simulink model "SingleTankOnOffControl_sim"  (R2021a)
settings: Solver=FixedStepAuto  StartTime=0.0  StopTime=40  FixedStep=0.1  RelTol=1e-3
InitFcn:
  | clearvars;
  | load('singletank_parameters.mat')
StopFcn:
  | plot_results
values from neighbouring files (symbols this model uses):
  params_single =     [singletank_parameters.mat]
libraries: simulink x1
settings Model: Creator=ksto036  LastModifiedBy=bl4ck
settings SolverCC: AlgebraicLoopSolver=TrustRegion
settings DataIOCC: SaveOutput=off  SignalLogging=off  DSMLogging=off  SaveTime=off  ReturnWorkspaceOutputs=off
settings DebuggingCC: SFMachineParentedDataDiag=warning

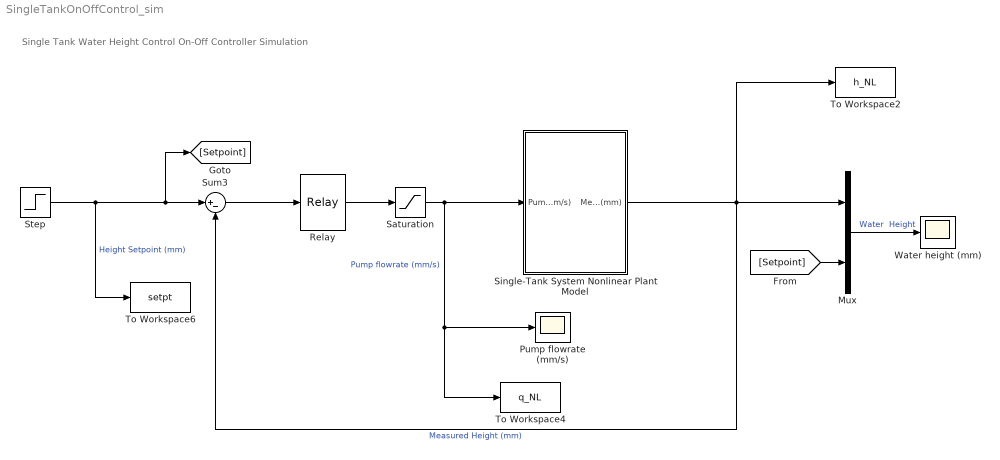
== system SingleTankOnOffControl_sim ==
  note: Single Tank Water Height Control
      | On-Off Controller
      | Simulation
  " Single-Tank System Nonlinear Plant Model" : Subsystem
      mask Display: image('$imagefile'); % Use "Edit Image" on toolstrip to change.
  Mux : Mux  Inputs=2
  Pump flowrate (mm/s) : Scope
  Relay : Relay  OnSwitchValue=3  OffSwitchValue=-3  OnOutputValue=params_single.Qlimit
  Saturation : Saturate  UpperLimit=params_single.Qlimit  LowerLimit=0  LinearizeAsGain=off
  Step : Step  Time=0  After=150  SampleTime=0
  Sum3 : Sum  Inputs=|+-
  To Workspace2 : ToWorkspace  VariableName=h_NL  SaveFormat=Structure With Time  SampleTime=-1
  To Workspace4 : ToWorkspace  VariableName=q_NL  SaveFormat=Structure With Time  SampleTime=-1
  To Workspace6 : ToWorkspace  VariableName=setpt  SaveFormat=Structure With Time  SampleTime=-1
  Water height (mm) : Scope
  wires:
  Step/1 -> [Setpoint], Sum3/1, To Workspace6/1  "Height Setpoint (mm)"
  Mux/1 -> Water height (mm)/1  "Water  Height"
  Sum3/1 -> Relay/1
  Saturation/1 -> " Single-Tank System Nonlinear Plant Model"/1(Pump Flowrate (mm/s)), Pump flowrate (mm/s)/1, To Workspace4/1  "Pump flowrate (mm/s)"
  Relay/1 -> Saturation/1
  " Single-Tank System Nonlinear Plant Model"/1(Measured Height (mm)) -> Mux/1, To Workspace2/1, Sum3/2  "Measured Height (mm)"
  [Setpoint] -> Mux/2

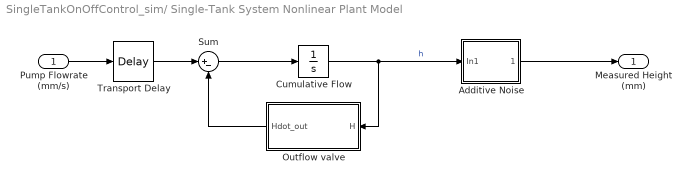
== system SingleTankOnOffControl_sim/ Single-Tank System Nonlinear Plant Model ==
  Pump Flowrate (mm/s) : Inport
  Additive Noise : Subsystem
  Cumulative Flow : Integrator  LimitOutput=on  UpperSaturationLimit=params_single.Hlimit  LowerSaturationLimit=0
  Outflow valve : Subsystem
  Sum : Sum  Inputs=|+-
  Transport Delay : TransportDelay
  Measured Height (mm) : Outport  VectorParamsAs1DForOutWhenUnconnected=off
  wires:
  Sum/1 -> Cumulative Flow/1
  Cumulative Flow/1 -> Additive Noise/1(In1), Outflow valve/1(H)  "h"
  Outflow valve/1(Hdot_out) -> Sum/2
  Additive Noise/1(Measured Height (mm)) -> Measured Height (mm)/1
  Pump Flowrate (mm/s)/1 -> Transport Delay/1
  Transport Delay/1 -> Sum/1

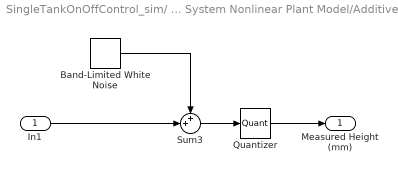
== system SingleTankOnOffControl_sim/ Single-Tank System Nonlinear Plant Model/Additive Noise ==
  In1 : Inport
  Band-Limited White Noise : simulink/Sources/Band-Limited White Noise  Cov=[0.01]  Ts=0.1  seed=[23341]
  Quantizer : Quantizer  QuantizationInterval=0.2
  Sum3 : Sum  Inputs=++|  SaturateOnIntegerOverflow=on
  Measured Height (mm) : Outport  VectorParamsAs1DForOutWhenUnconnected=off
  wires:
  In1/1 -> Sum3/2
  Sum3/1 -> Quantizer/1
  Band-Limited White Noise/1 -> Sum3/1
  Quantizer/1 -> Measured Height (mm)/1

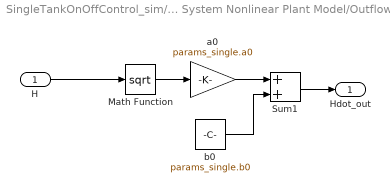
== system SingleTankOnOffControl_sim/ Single-Tank System Nonlinear Plant Model/Outflow valve ==
  H : Inport
  Math Function : Math  Operator=sqrt  SignedPower=on  SaturateOnIntegerOverflow=on
  Sum1 : Sum  SaturateOnIntegerOverflow=on
  a0 : Gain  Gain=params_single.a0  SaturateOnIntegerOverflow=on  OutDataTypeStr=Inherit: Same as input  ParamDataTypeStr=Inherit: Same as input
  b0 : Constant  Value=params_single.b0
  Hdot_out : Outport  VectorParamsAs1DForOutWhenUnconnected=off
  wires:
  b0/1 -> Sum1/2
  Sum1/1 -> Hdot_out/1
  H/1 -> Math Function/1
  a0/1 -> Sum1/1
  Math Function/1 -> a0/1
